simulink model "Task1_ScientificCalculator"  (R2021a)
settings: Solver=FixedStepDiscrete  StartTime=0.0  StopTime=10.0  RelTol=1e-3  EnableMultiTasking=on
settings Model: SILPILModeSetting=veronly  ExtModeTrigDuration=2  Creator=Michael_Ibrahim  LastModifiedBy=Michael_Ibrahim
settings DataIOCC: ReturnWorkspaceOutputs=off
settings OptimizationCC: EnableMemcpy=off  LifeSpan=1  MaxStackSize=64  EfficientTunableParamExpr=on
settings DebuggingCC: UnderspecifiedInitializationDetection=Classic  MergeDetectMultiDrivingBlocksExec=none  SFMachineParentedDataDiag=warning  ArithmeticOperatorsInVariantConditions=warning
settings HardwareCC: ProdBitPerInt=16  ProdBitPerPointer=16  ProdBitPerSizeT=16  ProdBitPerPtrDiffT=16  ProdLargestAtomicFloat=None  ProdWordSize=8  ProdHWDeviceType=Atmel->AVR
settings ModelReferenceCC: PropagateSignalLabelsOutOfModel=off
settings SFSimCC: MATLABDynamicMemAlloc=off  CustomCodeUndefinedFunction=UseInterfaceOnly
settings RTWCC: SystemTargetFile=ert.tlc  HardwareBoard=Arduino Uno  GenCodeOnly=on  TemplateMakefile=ert_default_tmf  GenerateReport=on  Toolchain=Arduino AVR  IncludeHyperlinkInReport=on  LaunchReport=on  GenerateTraceInfo=on  GenerateTraceReport=on  GenerateTraceReportSl=on  GenerateTraceReportSf=on  GenerateTraceReportEml=on
settings CodeAppCC: ForceParamTrailComments=on  IgnoreCustomStorageClasses=off  OperatorAnnotations=on  SimulinkDataObjDesc=on  SFDataObjDesc=on  MATLABFcnDesc=on  InsertBlockDesc=on  StateflowObjectComments=on  MATLABSourceComments=on
settings ERTTargetCC: MultiwordLength=2048  SupportContinuousTime=on  SupportVariableSizeSignals=on  ExtModeStaticAllocSize=250

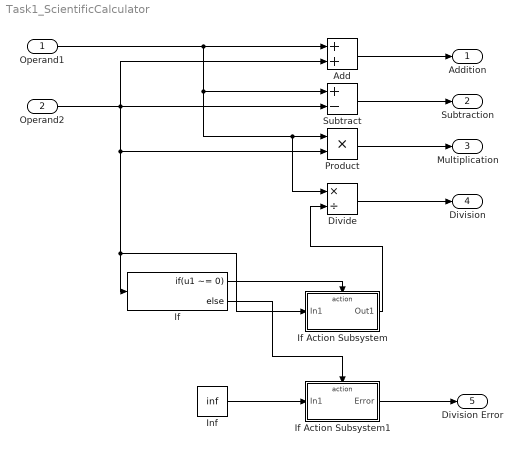
== system Task1_ScientificCalculator ==
  Operand1 : Inport
  Operand2 : Inport  Port=2
  Add : Sum
  Divide : Product  Inputs=*/
  If : If  IfExpression=u1 ~= 0
  If Action Subsystem : Subsystem  TreatAsAtomicUnit=on
  If Action Subsystem1 : Subsystem  TreatAsAtomicUnit=on
  Inf : Constant  Value=inf
  Product : Product
  Subtract : Sum  Inputs=+-
  Addition : Outport
  Subtraction : Outport  Port=2
  Multiplication : Outport  Port=3
  Division : Outport  Port=4
  Division Error : Outport  Port=5
  wires:
  Operand1/1 -> Divide/1, Product/1, Subtract/1, Add/1
  If/1 -> If Action Subsystem/Action
  Operand2/1 -> If/1, If Action Subsystem/1(In1), Product/2, Subtract/2, Add/2
  If Action Subsystem/1(Out1) -> Divide/2
  If/2 -> If Action Subsystem1/Action
  Divide/1 -> Division/1
  Inf/1 -> If Action Subsystem1/1(In1)
  Subtract/1 -> Subtraction/1
  Add/1 -> Addition/1
  Product/1 -> Multiplication/1
  If Action Subsystem1/1(Error) -> Division Error/1

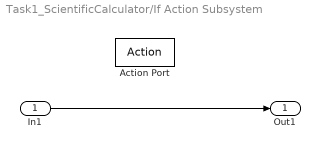
== system Task1_ScientificCalculator/If Action Subsystem ==
  In1 : Inport
  Action Port : ActionPort  ActionPortLabel=if(u1 ~= 0)
  Out1 : Outport
  wires:
  In1/1 -> Out1/1

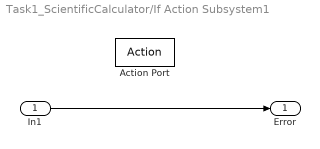
== system Task1_ScientificCalculator/If Action Subsystem1 ==
  In1 : Inport
  Action Port : ActionPort  ActionPortLabel=else
  Error : Outport
  wires:
  In1/1 -> Error/1
